simulink model "untitled"  (R2013b)
settings: Solver=FixedStepDiscrete  StartTime=0.0  StopTime=80  FixedStep=0.002  RelTol=1e-3
libraries: simulink x2
settings Model: Creator=mwegiere  LastModifiedBy=mwegiere

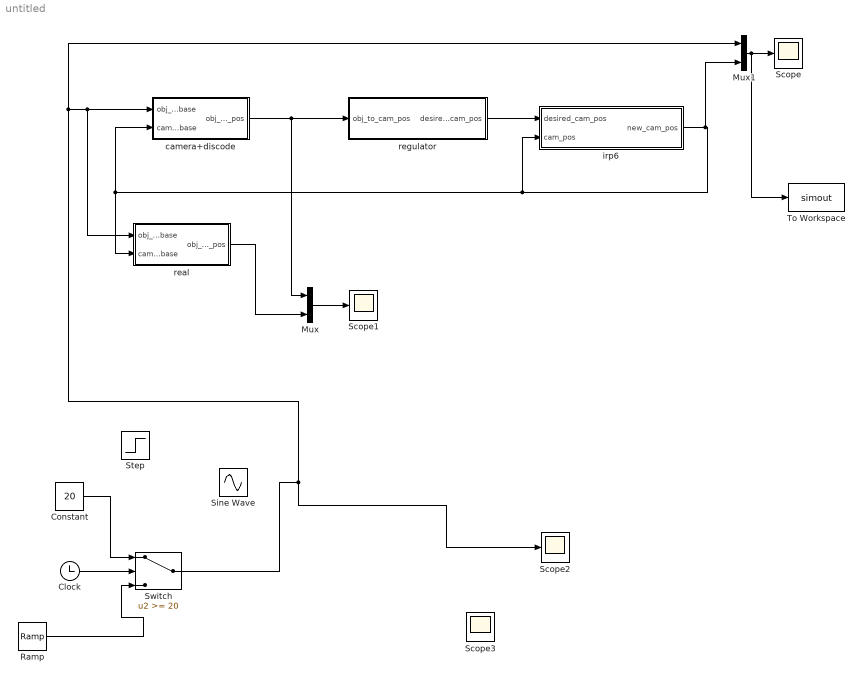
== system untitled ==
  Clock : Clock
  Constant : Constant  Value=20
  Mux : Mux  Inputs=2
  Mux1 : Mux  Inputs=2
  Ramp : simulink/Sources/Ramp  slope=1  start=0  X0=0
  Scope{,1..3} (4 alike) : Scope
      Scope1 settings: TimeRange=60  YMin=-2  YMax=3
      Scope2 settings: TimeRange=3  SaveName=ScopeData2
      Scope3 settings: TimeRange=3  SaveName=ScopeData3
  Sine Wave : Sin  SampleTime=0
  Step : Step  SampleTime=0
  Switch : Switch  Threshold=20
  To Workspace : ToWorkspace  VariableName=simout  SampleTime=-1  SaveFormat=Timeseries
  camera+discode : Subsystem
  irp6 : Subsystem
  "real " : Subsystem
  regulator : Subsystem
  wires:
  Switch/1 -> Scope2/1, Mux1/1, camera+discode/1(obj_pos_base), "real "/1(obj_pos_base)
  irp6/1("new_cam_pos ") -> Mux1/2, irp6/2("cam_pos "), "real "/2(cam_pos_base), camera+discode/2(cam_pos_base)
  regulator/1(desired_cam_pos) -> irp6/1("desired_cam_pos ")
  camera+discode/1(obj_to_cam_pos) -> Mux/1, regulator/1(obj_to_cam_pos)
  Mux/1 -> Scope1/1
  "real "/1(obj_to_cam_pos) -> Mux/2
  Mux1/1 -> To Workspace/1, Scope/1
  Clock/1 -> Switch/2
  Constant/1 -> Switch/1
  Ramp/1 -> Switch/3

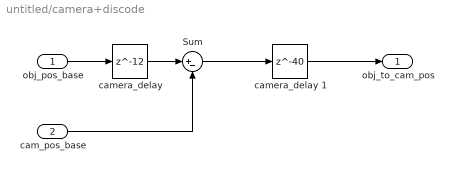
== system untitled/camera+discode ==
  obj_pos_base : Inport
  cam_pos_base : Inport  Port=2
  " camera_delay " : Delay  DelayLength=12
  " camera_delay 1" : Delay  DelayLength=40
  Sum : Sum  Inputs=|+-
  obj_to_cam_pos : Outport
  wires:
  cam_pos_base/1 -> Sum/2
  obj_pos_base/1 -> " camera_delay "/1
  Sum/1 -> " camera_delay 1"/1
  " camera_delay "/1 -> Sum/1
  " camera_delay 1"/1 -> obj_to_cam_pos/1

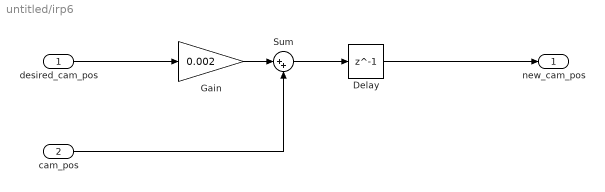
== system untitled/irp6 ==
  "desired_cam_pos " : Inport
  "cam_pos " : Inport  Port=2
  Delay : Delay  DelayLength=1  InitialCondition=0
  Gain : Gain  Gain=0.002
  Sum : Sum  Inputs=|++
  "new_cam_pos " : Outport
  wires:
  Delay/1 -> "new_cam_pos "/1
  "desired_cam_pos "/1 -> Gain/1
  "cam_pos "/1 -> Sum/2
  Gain/1 -> Sum/1
  Sum/1 -> Delay/1

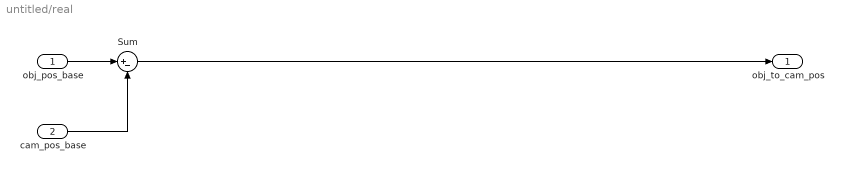
== system untitled/real  ==
  obj_pos_base : Inport
  cam_pos_base : Inport  Port=2
  Sum : Sum  Inputs=|+-
  obj_to_cam_pos : Outport
  wires:
  Sum/1 -> obj_to_cam_pos/1
  obj_pos_base/1 -> Sum/1
  cam_pos_base/1 -> Sum/2

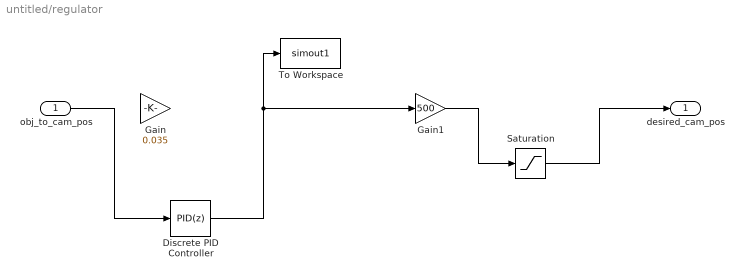
== system untitled/regulator ==
  obj_to_cam_pos : Inport
  Discrete PID Controller : simulink/Continuous/PID Controller  Controller=PID  TimeDomain=Discrete-time  SampleTime=-1  IntegratorMethod=Forward Euler  FilterMethod=Forward Euler  Form=Parallel  P=0.0023947713404702  I=2.10507979851124e-05  D=-0.0012485808414782  N=1.4202345593281  InitialConditionSource=internal  InitialConditionForIntegrator=0  InitialConditionForFilter=0  ExternalReset=none  LimitOutput=off  UpperSaturationLimit=inf  LowerSaturationLimit=-inf  LinearizeAsGain=off  AntiWindupMode=none  Kb=1  TrackingMode=off  Kt=1  PParamMin=[]  PParamMax=[]  IParamMin=[]  IParamMax=[]  DParamMin=[]  DParamMax=[]  NParamMin=[]  NParamMax=[]  KbParamMin=[]  KbParamMax=[]  KtParamMin=[]  KtParamMax=[]  POutMin=[]  POutMax=[]  IOutMin=[]  IOutMax=[]  DOutMin=[]  DOutMax=[]  NOutMin=[]  NOutMax=[]  KbOutMin=[]  KbOutMax=[]  KtOutMin=[]  KtOutMax=[]  IntegratorOutMin=[]  IntegratorOutMax=[]  FilterOutMin=[]  FilterOutMax=[]  SumOutMin=[]  SumOutMax=[]  SumI1OutMin=[]  SumI1OutMax=[]  SumI2OutMin=[]  SumI2OutMax=[]  SumI3OutMin=[]  SumI3OutMax=[]  SumDOutMin=[]  SumDOutMax=[]  SaturationOutMin=[]  SaturationOutMax=[]  IntegratorContinuousStateAttributes=''  IntegratorStateMustResolveToSignalObject=off  IntegratorRTWStateStorageClass=Auto  FilterContinuousStateAttributes=''  FilterStateMustResolveToSignalObject=off  FilterRTWStateStorageClass=Auto
  Gain : Gain  Gain=0.035
  Gain1 : Gain  Gain=500
  Saturation : Saturate  UpperLimit=10  LowerLimit=-10
  To Workspace : ToWorkspace  VariableName=simout1  SampleTime=-1  SaveFormat=Timeseries
  desired_cam_pos : Outport
  wires:
  obj_to_cam_pos/1 -> Discrete PID Controller/1
  Discrete PID Controller/1 -> To Workspace/1, Gain1/1
  Gain1/1 -> Saturation/1
  Saturation/1 -> desired_cam_pos/1
